simulink model "step_ramp_demo"  (R2021a)
settings: Solver=VariableStepAuto  StartTime=0.0  StopTime=10.0  RelTol=1e-3
undefined symbols (not defined in the file or in its folder): Jounce, Snap
libraries: ssrlib x2
settings Model: Creator=SESA564501  LastModifiedBy=sk

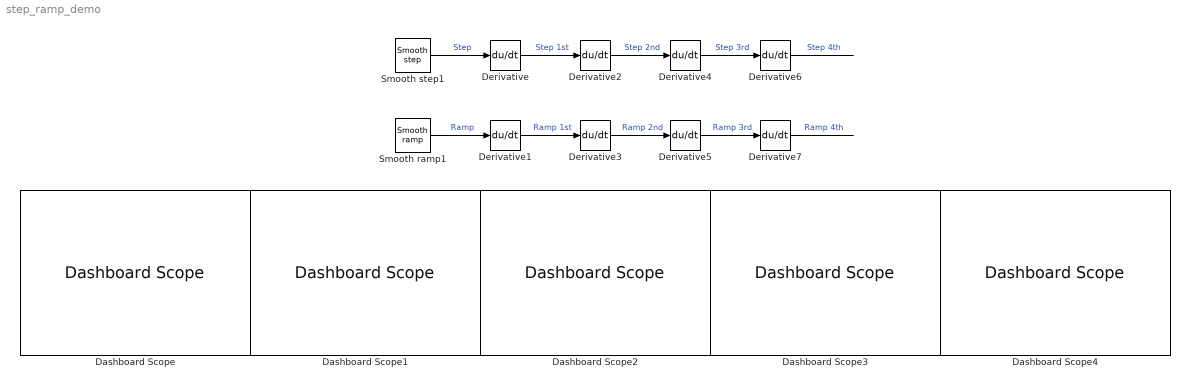
== system step_ramp_demo ==
  Dashboard Scope{,1..4} (5 alike) : DashboardScope
  Derivative{,1..7} (8 alike) : Derivative
  Smooth ramp1 : ssrlib/Smooth ramp  startTime=5  endTime=8  startValue=1  Slope=2  Smoothness=Snap/Jounce (4)
  Smooth step1 : ssrlib/Smooth step  startTime=1  endTime=6  startValue=2  endValue=5  Smoothness=Snap/Jounce (4)
  wires:
  Smooth step1/1 -> Derivative/1  "Step"
  Smooth ramp1/1 -> Derivative1/1  "Ramp"
  Derivative/1 -> Derivative2/1  "Step 1st"
  Derivative1/1 -> Derivative3/1  "Ramp 1st"
  Derivative3/1 -> Derivative5/1  "Ramp 2nd"
  Derivative2/1 -> Derivative4/1  "Step 2nd"
  Derivative4/1 -> Derivative6/1  "Step 3rd"
  Derivative5/1 -> Derivative7/1  "Ramp 3rd"
  Derivative6/1 -> ?  "Step 4th"
  Derivative7/1 -> ?  "Ramp 4th"
